simulink library "rllib"  (R2020a)
settings: Solver=VariableStepAuto  StartTime=0.0  StopTime=10.0  RelTol=1e-3
undefined symbols (not defined in the file or in its folder): agentObj, getSampleTime
settings Model: Creator=The MathWorks, Inc.  LastModifiedBy=The MathWorks, Inc.
settings DataIOCC: ReturnWorkspaceOutputs=off
settings DebuggingCC: ArithmeticOperatorsInVariantConditions=warning
settings SFSimCC: SimUseLocalCustomCode=off  CustomCodeUndefinedFunction=UseInterfaceOnly
settings RTWCC: RTWUseLocalCustomCode=off

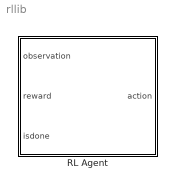
== system rllib ==
  RL Agent : Subsystem  mask(RL Agent){Agent=agentObj, ProvideReward=on, ProvideIsDone=on, ProvideCumRwd=off, TreatAsDirectFeedthrough=on, CollectLoggedSignals=on, CollectModelStates=on}
      mask prompts: Agent "rl:block:RLAgentAgentPrompt"; ProvideReward "rl:block:RLAgentProvideRewardPrompt"; ProvideIsDone "rl:block:RLAgentProvideIsDonePrompt"; ProvideCumRwd "rl:block:RLAgentProvideCumRwdPrompt"; TreatAsDirectFeedthrough "rl:block:RLAgentDirectFeedthroughPrompt"; CollectLoggedSignals "rl:block:RLAgentCollectLoggedSignalsPrompt"; CollectModelStates "rl:block:RLAgentCollectModelStatesPrompt"
      mask help: rl:block:RLAgentDescription
      mask init:
      | rl.simulink.blocks.agentmaskinit(gcb);
      mask Help: eval('rl.util.guihelp(''rlAgentBlock'')')
      mask DialogControl BDCollapsible Prompt: Block Diagram
      mask DialogControl AgentGroup Prompt: rl:block:RLAgentAgentGroupPrompt
      mask DialogControl Agent Prompt: Agent object
      mask DialogControl Agent Tooltip: rl:block:RLAgentAgentTooltip
      mask DialogControl PortGroup Prompt: rl:block:RLAgentPortsGroupPrompt
      mask DialogControl ProvideReward Prompt: Provide reward signal
      mask DialogControl ProvideReward Tooltip: rl:block:RLAgentProvideRewardTooltip
      mask DialogControl ProvideIsDone Prompt: Provide isdone signal
      mask DialogControl ProvideIsDone Tooltip: rl:block:RLAgentProvideIsDoneTooltip
      mask DialogControl ProvideCumRwd Prompt: Output cumulative reward signal
      mask DialogControl ProvideCumRwd Tooltip: rl:block:RLAgentProvideCumRwdTooltip
      mask DialogControl DirectFeedThroughGroup Prompt: rl:block:RLAgentDirectFeedthroughGroupPrompt
      mask DialogControl TreatAsDirectFeedthrough Prompt: Treat inputs as direct feedthrough
      mask DialogControl TreatAsDirectFeedthrough Tooltip: rl:block:RLAgentDirectFeedthroughTooltip
      mask DialogControl DataGroup Prompt: rl:block:RLAgentDataGroupPrompt
      mask DialogControl CollectLoggedSignals Prompt: Provide logged signals to agent
      mask DialogControl CollectLoggedSignals Tooltip: rl:block:RLAgentCollectLoggedSignalsTooltip
      mask DialogControl CollectModelStates Prompt: Provide model states to agent
      mask DialogControl CollectModelStates Tooltip: rl:block:RLAgentCollectModelStatesTooltip

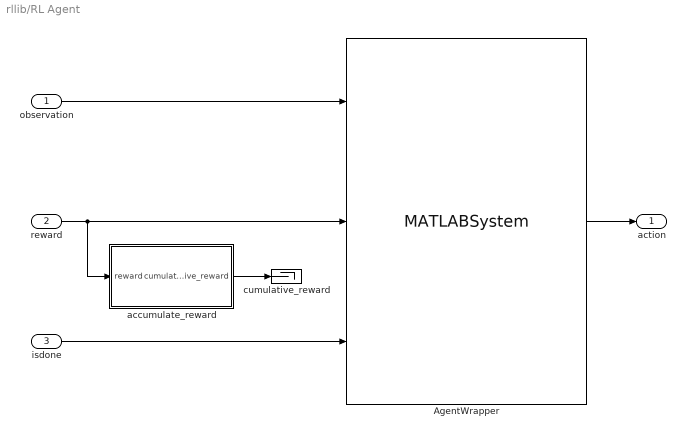
== system rllib/RL Agent ==
  observation : Inport
  reward : Inport  Port=2
  isdone : Inport  Port=3
  AgentWrapper : MATLABSystem  System=rl.simulink.blocks.AgentWrapper  ModelName=rllib  AgentObjectName=Agent  BlockPath=rllib/RL Agent/AgentWrapper  TreatAsDirectFeedthrough=true  IsRewardProvided=true  IsIsDoneProvided=true  CollectLoggedSignals=true  CollectModelStates=true
      mask Type: rl.simulink.blocks.AgentWrapper
      mask Display:
      | disp('AgentWrapper');
      | port_label('input',1,'observation');
      | port_label('input',2,'reward');
      | port_label('input',3,'isdone');
      | port_label('output',1,'action');
  accumulate_reward : Subsystem
  cumulative_reward : Terminator
      settings: BlockKeywords=__PRM__SERIALIZED__DATA__:End,Simulink:BlockKeywords:Sinks_Terminator_Terminator,Simulink:BlockKeywords:Sinks_Terminator_End
  action : Outport  VectorParamsAs1DForOutWhenUnconnected=off
  wires:
  observation/1 -> AgentWrapper/1
  AgentWrapper/1 -> action/1
  reward/1 -> accumulate_reward/1(reward), AgentWrapper/2
  isdone/1 -> AgentWrapper/3
  accumulate_reward/1(cumulative_reward) -> cumulative_reward/1

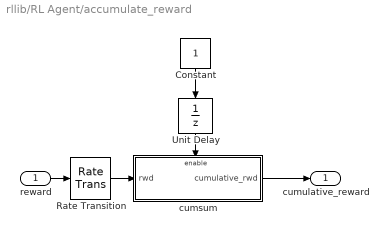
== system rllib/RL Agent/accumulate_reward ==
  reward : Inport
  Constant : Constant
  Rate Transition : RateTransition  OutPortSampleTime=getSampleTime(Agent)
  Unit Delay : UnitDelay  SampleTime=-1  HasFrameUpgradeWarning=on
  cumsum : Subsystem
  cumulative_reward : Outport  VectorParamsAs1DForOutWhenUnconnected=off
  wires:
  cumsum/1(cumulative_rwd) -> cumulative_reward/1
  Unit Delay/1 -> cumsum/Enable
  Constant/1 -> Unit Delay/1
  reward/1 -> Rate Transition/1
  Rate Transition/1 -> cumsum/1(rwd)

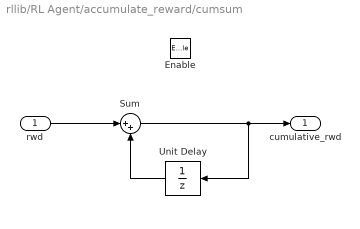
== system rllib/RL Agent/accumulate_reward/cumsum ==
  rwd : Inport
  Enable : EnablePort
  Sum : Sum  Inputs=|++
  Unit Delay : UnitDelay  SampleTime=-1  HasFrameUpgradeWarning=on
  cumulative_rwd : Outport  VectorParamsAs1DForOutWhenUnconnected=off
  wires:
  rwd/1 -> Sum/1
  Sum/1 -> Unit Delay/1, cumulative_rwd/1
  Unit Delay/1 -> Sum/2
